simulink model "Respiratory"  (Simulink 6.4)
settings: Solver=ode45  StartTime=0.0  StopTime=10.0  RelTol=1e-3
values from neighbouring files (symbols this model uses):
  a1 = 0.3836    [Dissociation_Spencer_IC.m]    (also in Gas_Exchange_IC.m; Respiratory_IC.m)
  a2 = 1.819    [Dissociation_Spencer_IC.m]    (also in Gas_Exchange_IC.m; Respiratory_IC.m)
  alpha1 = 0.02598    [Dissociation_Spencer_IC.m]    (also in Gas_Exchange_IC.m; Respiratory_IC.m)
  alpha2 = 0.05591    [Dissociation_Spencer_IC.m]    (also in Gas_Exchange_IC.m; Respiratory_IC.m)
  beta1 = 0.012275    [Dissociation_Spencer_IC.m]    (also in Gas_Exchange_IC.m; Respiratory_IC.m)
  beta2 = 0.03255    [Dissociation_Spencer_IC.m]    (also in Gas_Exchange_IC.m; Respiratory_IC.m)
  C1 = 9    [Dissociation_Spencer_IC.m]    (also in Gas_Exchange_IC.m; Respiratory_IC.m)
  C2 = 87.00    (= 87)    [Dissociation_Spencer_IC.m]    (also in Gas_Exchange_IC.m; Respiratory_IC.m)
  Circadian_Period = 24    [Respiratory_IC.m]    (also in State_UA_Khoo_IC.m)
  CvCO2IC = 0.5116    [Body_Khoo_IC.m]    (also in Gas_Exchange_IC.m; Respiratory_IC.m = 0.5247)
  CvO2IC = 0.1672    [Body_Khoo_IC.m]    (also in Gas_Exchange_IC.m; Respiratory_IC.m = 0.1639)
  Dead1CO2IC = 0.1020    (= 0.102)    [Dead_Space_Khoo_IC.m]    (also in Gas_Exchange_IC.m; Respiratory_IC.m = 39.5616)
  Dead1O2IC = 149.8824    [Dead_Space_Khoo_IC.m]    (also in Gas_Exchange_IC.m; Respiratory_IC.m = 104.3637)
  Dead2CO2IC = 0.5274    [Dead_Space_Khoo_IC.m]    (also in Gas_Exchange_IC.m; Respiratory_IC.m = 39.6736)
  Dead2O2IC = 149.3923    [Dead_Space_Khoo_IC.m]    (also in Gas_Exchange_IC.m; Respiratory_IC.m = 104.2258)
  Dead3CO2IC = 2.2996    [Dead_Space_Khoo_IC.m]    (also in Gas_Exchange_IC.m; Respiratory_IC.m = 39.8127)
  Dead3O2IC = 147.3503    [Dead_Space_Khoo_IC.m]    (also in Gas_Exchange_IC.m; Respiratory_IC.m = 104.0505)
  Dead4CO2IC = 8.2293    [Dead_Space_Khoo_IC.m]    (also in Gas_Exchange_IC.m; Respiratory_IC.m = 40.0061)
  Dead4O2IC = 140.5179    [Dead_Space_Khoo_IC.m]    (also in Gas_Exchange_IC.m; Respiratory_IC.m = 103.8005)
  Dead5CO2IC = 22.0757    [Dead_Space_Khoo_IC.m]    (also in Gas_Exchange_IC.m; Respiratory_IC.m = 40.3359)
  Dead5O2IC = 124.5641    [Dead_Space_Khoo_IC.m]    (also in Gas_Exchange_IC.m; Respiratory_IC.m = 103.3579)
  E_CW = 5    [Pleural_Schuessler_IC.m]    (also in Pmus_Flow_Younes_IC.m; Resp_Mech_IC.m; Respiratory_IC.m)
  E_L = 5    [Pleural_Schuessler_IC.m]    (also in Pmus_Flow_Younes_IC.m; Resp_Mech_IC.m; Respiratory_IC.m)
  fc = 0.4/60    (= 0.00666666666667)    [Respiratory_IC.m]    (also in State_UA_Khoo_IC.m)
  FlowIC = 0    [Pmus_Flow_Younes_IC.m]    (also in Resp_Mech_IC.m; Respiratory_IC.m)
  gc = 0.008/60    (= 0.000133333333333)    [Respiratory_IC.m]    (also in State_UA_Khoo_IC.m)
  h = 0.0183    [Brain_Khoo_IC.m]    (also in Gas_Exchange_IC.m; Respiratory_IC.m)
  K1 = 13    [Dissociation_Spencer_IC.m]    (also in Gas_Exchange_IC.m; Respiratory_IC.m)
  K2 = 194.4    [Dissociation_Spencer_IC.m]    (also in Gas_Exchange_IC.m; Respiratory_IC.m)
  MRbCO2 = 0.0517    [Brain_Khoo_IC.m]    (also in Gas_Exchange_IC.m; Respiratory_IC.m)
  MRCO2 = 0.0033    [Body_Khoo_IC.m]    (also in Gas_Exchange_IC.m; Respiratory_IC.m)
  MRO2 = 0.0038    [Body_Khoo_IC.m]    (also in Gas_Exchange_IC.m; Respiratory_IC.m)
  PACO2_delayIC = 39.6041    [Cardio_Mix_Lange_IC.m]    (also in Gas_Exchange_IC.m; Respiratory_IC.m = 40.4448)
  PaCO2firstIC = 0.2150    (= 0.215)    [Cardio_Mix_Lange_IC.m]    (also in Gas_Exchange_IC.m; Respiratory_IC.m = -0.2465)
  PACO2IC = 37.1484    [Gas_Exchange_IC.m]    (also in Lungs_Khoo_IC.m; Respiratory_IC.m = 40.9432)
  PaCO2secondIC = 38.4577    [Cardio_Mix_Lange_IC.m]    (also in Gas_Exchange_IC.m; Respiratory_IC.m = 40.3928)
  PAO2_delayIC = 103.8436    [Cardio_Mix_Lange_IC.m]    (also in Gas_Exchange_IC.m; Respiratory_IC.m = 103.1223)
  PaO2firstIC = -0.2838    [Cardio_Mix_Lange_IC.m]    (also in Gas_Exchange_IC.m; Respiratory_IC.m = 0.3557)
  PAO2IC = 107.1983    [Gas_Exchange_IC.m]    (also in Lungs_Khoo_IC.m; Respiratory_IC.m = 102.5153)
  PaO2secondIC = 105.4828    [Cardio_Mix_Lange_IC.m]    (also in Gas_Exchange_IC.m; Respiratory_IC.m = 103.1435)
  PbCO2IC = 48.2858    [Brain_Khoo_IC.m]    (also in Gas_Exchange_IC.m; Respiratory_IC.m = 48.5383)
  PICO2 = 0    [Dead_Space_Khoo_IC.m]    (also in Gas_Exchange_IC.m; Respiratory_IC.m)
  PICO2_change = 0    [Respiratory_IC.m]
  PIO2 = 150    [Dead_Space_Khoo_IC.m]    (also in Gas_Exchange_IC.m; Respiratory_IC.m)
  PIO2_change = -90    [Mech_vent_test.m]    (also in Respiratory_IC.m = 0)
  Pt_frcIC1 = 0    [Pmus_Flow_Younes_IC.m]    (also in Resp_Mech_IC.m; Respiratory_IC.m)
  Pt_frcIC2 = 0    [Pmus_Flow_Younes_IC.m]    (also in Resp_Mech_IC.m; Respiratory_IC.m)
  QdBo = 0.8333    [Brain_Khoo_IC.m]    (also in Gas_Exchange_IC.m; Respiratory_IC.m)
  R_AW = 1.27    [Pleural_Schuessler_IC.m]    (also in Pmus_Flow_Younes_IC.m; Resp_Mech_IC.m; Respiratory_IC.m)
  R_CW = 1.03    [Pleural_Schuessler_IC.m]    (also in Pmus_Flow_Younes_IC.m; Resp_Mech_IC.m; Respiratory_IC.m)
  R_L = 1.69    [Pleural_Schuessler_IC.m]    (also in Pmus_Flow_Younes_IC.m; Resp_Mech_IC.m; Respiratory_IC.m)
  RC = 0.06    [Pleural_Schuessler_IC.m]    (also in Pmus_Flow_Younes_IC.m; Resp_Mech_IC.m; Respiratory_IC.m)
  rc = 0.2/60    (= 0.00333333333333)    [Respiratory_IC.m]    (also in State_UA_Khoo_IC.m)
  SbCO2 = 0.3600    (= 0.36)    [Brain_Khoo_IC.m]    (also in Gas_Exchange_IC.m; Respiratory_IC.m)
  SCO2 = 0.0043    [Brain_Khoo_IC.m]    (also in Gas_Exchange_IC.m; Respiratory_IC.m)
  SWAo = 0.007    [Respiratory_IC.m]    (also in State_UA_Khoo_IC.m)
  T1 = 1    [Cardio_Mix_Lange_IC.m]    (also in Gas_Exchange_IC.m; Respiratory_IC.m)
  T2 = 2    [Cardio_Mix_Lange_IC.m]    (also in Gas_Exchange_IC.m; Respiratory_IC.m)
  t_CO2_duration = 0    [Respiratory_IC.m]
  t_CO2_start = 0    [Respiratory_IC.m]
  t_end_UA = 0    [Respiratory_IC.m]    (also in State_UA_Khoo_IC.m)
  t_O2_duration = 0    [Mech_vent_test.m]    (also in Respiratory_IC.m)
  t_O2_start = 0    [Mech_vent_test.m]    (also in Respiratory_IC.m)
  t_start_UA = 0    [Respiratory_IC.m]    (also in State_UA_Khoo_IC.m)
  time_step = time_step    [acquire_data.m]    (also in acquire_data_save.m)
  VC = 5    [Pmus_Flow_Younes_IC.m]    (also in Resp_Mech_IC.m; Respiratory_IC.m)
  Vdead1 = 0.03    [Dead_Space_Khoo_IC.m]    (also in Gas_Exchange_IC.m; Respiratory_IC.m)
  Vdead2 = 0.03    [Dead_Space_Khoo_IC.m]    (also in Gas_Exchange_IC.m; Respiratory_IC.m)
  Vdead3 = 0.03    [Dead_Space_Khoo_IC.m]    (also in Gas_Exchange_IC.m; Respiratory_IC.m)
  Vdead4 = 0.03    [Dead_Space_Khoo_IC.m]    (also in Gas_Exchange_IC.m; Respiratory_IC.m)
  Vdead5 = 0.03    [Dead_Space_Khoo_IC.m]    (also in Gas_Exchange_IC.m; Respiratory_IC.m)
  VTCO2 = 15    [Body_Khoo_IC.m]    (also in Gas_Exchange_IC.m; Respiratory_IC.m)
  VtIC = 0    [Pmus_Flow_Younes_IC.m]    (also in Resp_Mech_IC.m; Respiratory_IC.m)
  VTO2 = 6    [Body_Khoo_IC.m]    (also in Gas_Exchange_IC.m; Respiratory_IC.m)
  Z = 0.0227    [Dissociation_Spencer_IC.m]    (also in Gas_Exchange_IC.m; Respiratory_IC.m)
undefined symbols (not defined in the file or in its folder): A_0_ua, Arousal_UAIC, b_ua, C_ua_awake, DAY, K_ua, R_LAW, R_trachea
libraries: simulink x1, simulink_extras x1
(part 1 of 2)
settings Model: LastModifiedBy=cPhonix
settings OptimizationCC: BlockReduction=off  BooleanDataType=off
settings DebuggingCC: SolverPrmCheckMsg=none  StrictBusMsg=None
settings HardwareCC: TargetUnknown=on

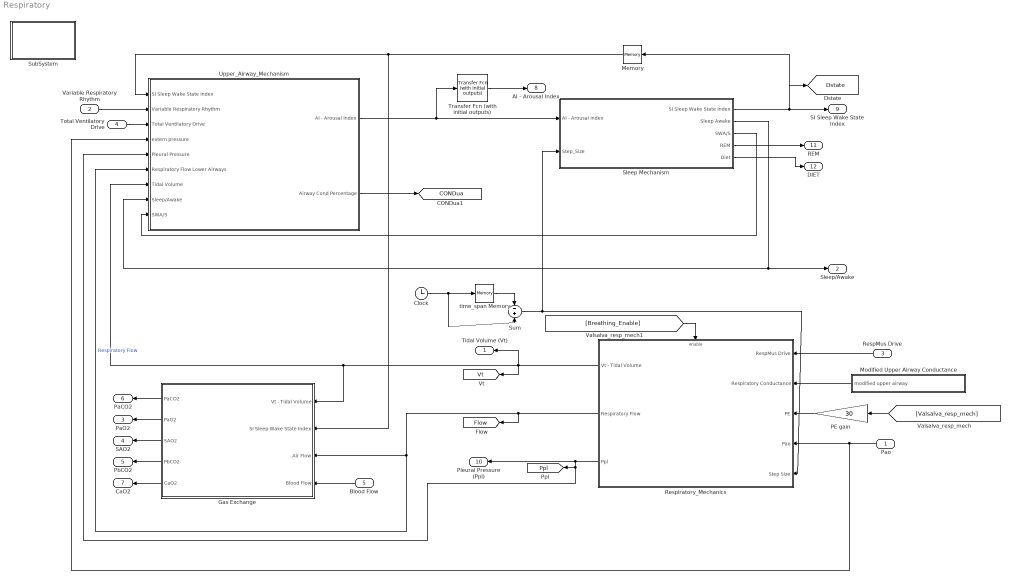
== system Respiratory ==
  Pao : Inport  Orientation=left
  Variable Respiratory Rhythm : Inport  Port=2
  RespMus Drive : Inport  Orientation=left  Port=3
  Total Ventilatory Drive : Inport  Port=4
  Blood Flow : Inport  Orientation=left  Port=5
  Clock : Clock
      settings: Decimation=10
  Gas Exchange : Subsystem  Orientation=left
  Memory : Memory  Orientation=left  InheritSampleTime=on
  Modified Upper Airway Conductance : Subsystem  Orientation=left
  PE gain : Gain  Orientation=left  Gain=30  SaturateOnIntegerOverflow=on
  Respiratory_Mechanics : Subsystem  Orientation=left  TreatAsAtomicUnit=on
      settings: PropExecContextOutsideSubsystem=on
  Sleep Mechanism : Subsystem
  SubSystem : Subsystem
      settings: OpenFcn=pneuma_variables
      mask Display: disp('"double click here"\n to load \nRespiratory \ninitial values');
  Sum : Sum  Inputs=-+  SaturateOnIntegerOverflow=on  InputSameDT=on
  Transfer Fcn (with initial outputs) : simulink_extras/Additional Linear/Transfer Fcn (with initial outputs)  SystemSampleTime=-1  N=1  D=[5 1]  Y0=Arousal_CardIC  U0=Arousal_CardIC
  Upper_Airway_Mechanism : Subsystem
  time_span Memory : Memory  X0=0-time_step
  Tidal Volume (Vt) : Outport  Orientation=left
  Sleep/Awake : Outport  Port=2
  PaO2 : Outport  Orientation=left  Port=3
  SAO2 : Outport  Orientation=left  Port=4
  PbCO2 : Outport  Orientation=left  Port=5
  PaCO2 : Outport  Orientation=left  Port=6
  CaO2 : Outport  Orientation=left  Port=7
  AI - Arousal Index : Outport  Port=8
  SI Sleep Wake State Index : Outport  Port=9
  Pleural Pressure (Ppl) : Outport  Orientation=left  Port=10
  REM : Outport  Port=11
  DIET : Outport  Port=12
  tag scope: CONDua=global, Dstate=global, Flow=global, Ppl=global, Vt=global
  wires:
  Respiratory_Mechanics/2(Respiratory Flow) -> Upper_Airway_Mechanism/6(Respiratory Flow Lower Airways), Gas Exchange/3(Air Flow), [Flow]  "Respiratory Flow"
  RespMus Drive/1 -> Respiratory_Mechanics/1("RespMus Drive ")
  PE gain/1 -> Respiratory_Mechanics/3("PE ")
  Total Ventilatory Drive/1 -> Upper_Airway_Mechanism/3(Total Ventilatory Drive)
  Modified Upper Airway Conductance/1(modified upper airway) -> Respiratory_Mechanics/2(Respiratory Conductance)
  Respiratory_Mechanics/1(Vt - Tidal Volume) -> Gas Exchange/1(Vt - Tidal Volume), Upper_Airway_Mechanism/7(Tidal Volume), Tidal Volume (Vt)/1, [Vt]
  Respiratory_Mechanics/3("Ppl ") -> Pleural Pressure (Ppl)/1, [Ppl], Upper_Airway_Mechanism/5(Pleural Pressure)
  Upper_Airway_Mechanism/1(AI - Arousal Index) -> Sleep Mechanism/1(AI - Arousal Index), Transfer Fcn (with initial outputs)/1
  Memory/1 -> Upper_Airway_Mechanism/1(SI Sleep Wake State Index), Gas Exchange/2(SI Sleep Wake State Index)
  Sleep Mechanism/1(SI Sleep Wake State Index) -> Memory/1, SI Sleep Wake State Index/1, [Dstate]
  Sleep Mechanism/2(Sleep Awake) -> Upper_Airway_Mechanism/8(Sleep/Awake), Sleep/Awake/1
  Upper_Airway_Mechanism/2("Airway Cond Percentage ") -> [CONDua]
  Gas Exchange/2(PaO2) -> PaO2/1
  Gas Exchange/1(PaCO2) -> PaCO2/1
  Gas Exchange/3(SAO2) -> SAO2/1
  Gas Exchange/4(PbCO2) -> PbCO2/1
  Pao/1 -> Upper_Airway_Mechanism/4(extern pressure), Respiratory_Mechanics/4("Pao ")
  Variable Respiratory Rhythm/1 -> Upper_Airway_Mechanism/2(Variable Respiratory Rhythm)
  Blood Flow/1 -> Gas Exchange/4(Blood Flow)
  [Breathing_Enable] -> Respiratory_Mechanics/Enable
  Sleep Mechanism/3(SWA/S) -> Upper_Airway_Mechanism/9(SWA/S)
  Clock/1 -> time_span Memory/1, Sum/2
  time_span Memory/1 -> Sum/1
  Sum/1 -> Respiratory_Mechanics/5(Step Size), Sleep Mechanism/2(Step_Size)
  Transfer Fcn (with initial outputs)/1 -> AI - Arousal Index/1
  Gas Exchange/5(CaO2) -> CaO2/1
  [Valsalva_resp_mech] -> PE gain/1
  Sleep Mechanism/4(REM) -> REM/1
  Sleep Mechanism/5(Diet) -> DIET/1

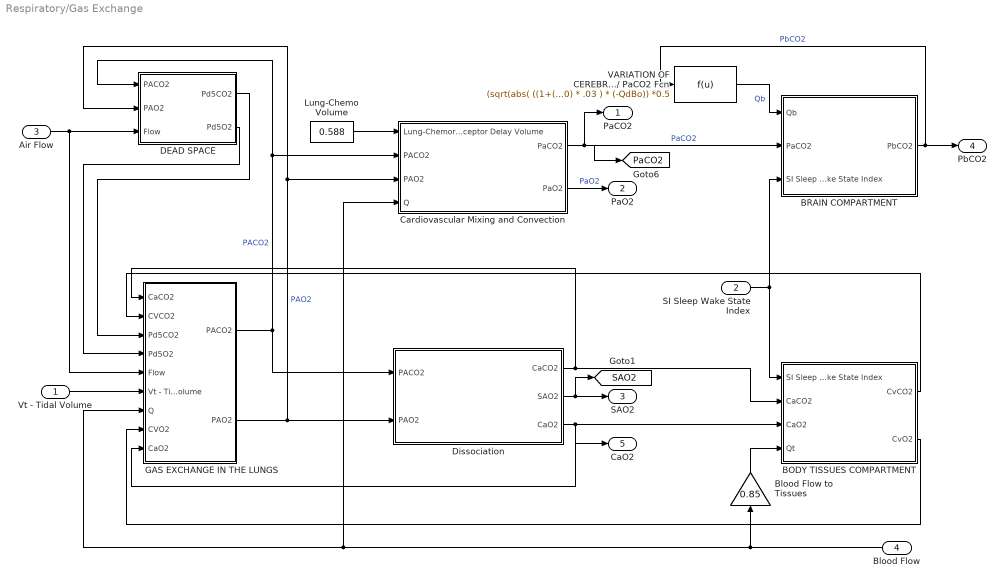
== system Respiratory/Gas Exchange ==
  Vt - Tidal Volume : Inport
  SI Sleep Wake State Index : Inport  Port=2
  Air Flow : Inport  Port=3
  Blood Flow : Inport  Orientation=left  Port=4
  BODY TISSUES COMPARTMENT : Subsystem
  BRAIN COMPARTMENT : Subsystem
  Blood Flow to Tissues : Gain  Orientation=up  Gain=0.85  SaturateOnIntegerOverflow=on
  Cardiovascular Mixing and Convection : Subsystem
  DEAD SPACE : Subsystem
  Dissociation : Subsystem
  GAS EXCHANGE IN THE LUNGS : Subsystem
  Lung-Chemo Volume : Constant  Value=0.588  OutDataType=sfix(16)  ConRadixGroup=Use specified scaling  OutScaling=2^0  SampleTime=inf  FramePeriod=inf
  VARIATION OF CEREBRAL BLOOD FLOW W/ PaCO2 Fcn : Fcn  Expr=(sqrt(abs( ((1+(u - 40) * .03 ) * (-QdBo))^2 - ( MRbCO2-h) * 4*0.03*QdBo/SCO2 ) )- (1+(u - 40) * .03 ) * (-QdBo)) *0.5
  PaCO2 : Outport
  PaO2 : Outport  Port=2
  SAO2 : Outport  Port=3
  PbCO2 : Outport  Port=4
  CaO2 : Outport  Port=5
  tag scope: PaCO2=global, SAO2=global
  wires:
  SI Sleep Wake State Index/1 -> BODY TISSUES COMPARTMENT/1(SI Sleep Wake State Index), BRAIN COMPARTMENT/3(SI Sleep Wake State Index)
  Cardiovascular Mixing and Convection/1(PaCO2) -> PaCO2/1, BRAIN COMPARTMENT/2(PaCO2), [PaCO2]  "PaCO2"
  BRAIN COMPARTMENT/1(PbCO2) -> PbCO2/1, VARIATION OF CEREBRAL BLOOD FLOW W/ PaCO2 Fcn/1  "PbCO2"
  DEAD SPACE/1(Pd5CO2) -> GAS EXCHANGE IN THE LUNGS/3(Pd5CO2)
  DEAD SPACE/2(Pd5O2) -> GAS EXCHANGE IN THE LUNGS/4(Pd5O2)
  GAS EXCHANGE IN THE LUNGS/2(PAO2) -> DEAD SPACE/2(PAO2), Cardiovascular Mixing and Convection/3(PAO2), Dissociation/2(PAO2)  "PAO2"
  Vt - Tidal Volume/1 -> GAS EXCHANGE IN THE LUNGS/6(Vt - Tidal Volume)
  Air Flow/1 -> DEAD SPACE/3(Flow), GAS EXCHANGE IN THE LUNGS/5(Flow)
  VARIATION OF CEREBRAL BLOOD FLOW W/ PaCO2 Fcn/1 -> BRAIN COMPARTMENT/1(Qb)  "Qb"
  GAS EXCHANGE IN THE LUNGS/1(PACO2) -> DEAD SPACE/1(PACO2), Cardiovascular Mixing and Convection/2(PACO2), Dissociation/1(PACO2)  "PACO2"
  Lung-Chemo Volume/1 -> Cardiovascular Mixing and Convection/1(Lung-Chemoreceptor Delay Volume)
  Blood Flow/1 -> Blood Flow to Tissues/1, GAS EXCHANGE IN THE LUNGS/7("Q "), Cardiovascular Mixing and Convection/4(Q)
  Cardiovascular Mixing and Convection/2(PaO2) -> PaO2/1  "PaO2"
  Blood Flow to Tissues/1 -> BODY TISSUES COMPARTMENT/4("Qt ")
  Dissociation/1(CaCO2) -> GAS EXCHANGE IN THE LUNGS/1(CaCO2), BODY TISSUES COMPARTMENT/2(CaCO2)
  Dissociation/3(CaO2) -> GAS EXCHANGE IN THE LUNGS/9(CaO2), CaO2/1, BODY TISSUES COMPARTMENT/3(CaO2)
  Dissociation/2(SAO2) -> [SAO2], SAO2/1
  BODY TISSUES COMPARTMENT/1(CvCO2) -> GAS EXCHANGE IN THE LUNGS/2(CVCO2)
  BODY TISSUES COMPARTMENT/2(CvO2) -> GAS EXCHANGE IN THE LUNGS/8(CVO2)

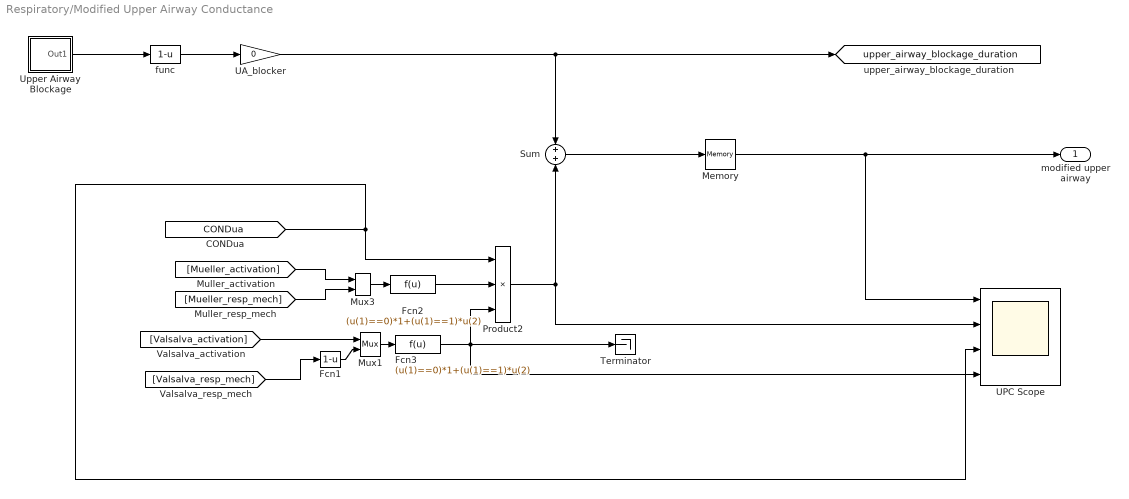
== system Respiratory/Modified Upper Airway Conductance ==
  Fcn1 : Fcn  Expr=1-u
  Fcn2 : Fcn  Expr=(u(1)==0)*1+(u(1)==1)*u(2)
  Fcn3 : Fcn  Expr=(u(1)==0)*1+(u(1)==1)*u(2)
  Memory : Memory
  Mux1 : Mux  Inputs=2
  Mux3 : Mux  Inputs=2
  Product2 : Product  Inputs=***  SaturateOnIntegerOverflow=on  InputSameDT=on
  Sum : Sum
  Terminator : Terminator
  UA_blocker : Gain  Gain=0  SaturateOnIntegerOverflow=on
  UPC Scope : Scope  NumInputPorts=4
      settings: TimeRange=120  YMin=-0.05~-0.05~0.4~-0.05  YMax=1.025~1.025~1.025~1.05  SaveName=ScopeData13  MaxDataPoints=50
  Upper Airway Blockage : Subsystem  mask{begin_time=t_start_UA, end_time=t_end_UA}
      mask prompts: begin_time "pulse begin"; end_time "pulse end"
      mask Display: disp('pulse')
  func : Fcn  Expr=1-u
  modified upper airway : Outport
  tag scope: upper_airway_blockage_duration=global
  wires:
  Upper Airway Blockage/1(Out1) -> func/1
  [Valsalva_resp_mech] -> Fcn1/1
  UA_blocker/1 -> [upper_airway_blockage_duration], Sum/1
  [CONDua] -> Product2/1, UPC Scope/3
  Product2/1 -> UPC Scope/2, Sum/2
  func/1 -> UA_blocker/1
  [Mueller_activation] -> Mux3/1
  [Mueller_resp_mech] -> Mux3/2
  Mux3/1 -> Fcn2/1
  Fcn2/1 -> Product2/2
  [Valsalva_activation] -> Mux1/1
  Mux1/1 -> Fcn3/1
  Fcn1/1 -> Mux1/2
  Fcn3/1 -> UPC Scope/4, Terminator/1, Product2/3
  Memory/1 -> modified upper airway/1, UPC Scope/1
  Sum/1 -> Memory/1

== system Respiratory/Respiratory_Mechanics ==
  "RespMus Drive " : Inport
  Respiratory Conductance : Inport  Port=2
  "PE " : Inport  Port=3
  "Pao " : Inport  Port=4
  Step Size : Inport  Port=5
  Enable : EnablePort  StatesWhenEnabling=reset  ZeroCross=off
  External Pressure Gain : Gain  Gain=0.1  SaturateOnIntegerOverflow=on
  Pleural Pressure Saturation : Saturate  UpperLimit=160  LowerLimit=-40  LinearizeAsGain=off  ZeroCross=off
  Pleural_Pressure1 : Subsystem
  Respiratory Muscles Activity1 : Subsystem
  Vt - Tidal Volume : Outport  InitialOutput=[0]
  Respiratory Flow : Outport  Port=2  InitialOutput=[0]
  "Ppl " : Outport  Port=3  InitialOutput=[0]
  wires:
  "PE "/1 -> Respiratory Muscles Activity1/2(PE)
  "RespMus Drive "/1 -> Respiratory Muscles Activity1/1(RespMus Drive)
  Respiratory Conductance/1 -> Respiratory Muscles Activity1/3("cond ")
  Respiratory Muscles Activity1/3(Pmus) -> Pleural_Pressure1/3(Pmus)
  "Pao "/1 -> External Pressure Gain/1
  External Pressure Gain/1 -> Pleural_Pressure1/4("Pao "), Respiratory Muscles Activity1/5(Pao)
  Respiratory Muscles Activity1/2(Vt) -> Pleural_Pressure1/2(Vt), Vt - Tidal Volume/1  "Vt Tidal Volume"
  Respiratory Muscles Activity1/1(Respiratory Flow) -> Pleural_Pressure1/1(Respiratory Flow), Respiratory Flow/1  "Flow"
  Step Size/1 -> Respiratory Muscles Activity1/4(Step Size)
  Pleural_Pressure1/1("Pleural Pressure (Ppl) ") -> Pleural Pressure Saturation/1
  Pleural Pressure Saturation/1 -> "Ppl "/1

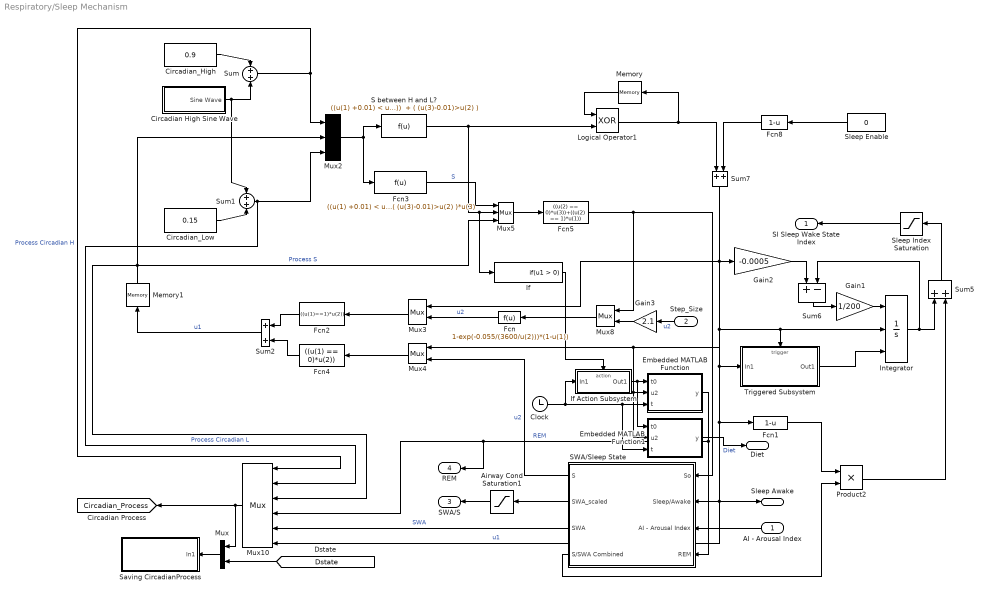
== system Respiratory/Sleep Mechanism ==
  AI - Arousal Index : Inport  Orientation=left
  Step_Size : Inport  Orientation=left  Port=2
  Airway Cond Saturation1 : Saturate  Orientation=left  UpperLimit=1  LowerLimit=0
  Circadian High Sine Wave : Subsystem
  Circadian_High : Constant  Value=0.9  OutDataType=sfix(16)  ConRadixGroup=Use specified scaling  OutScaling=2^0  SampleTime=inf  FramePeriod=inf
  Circadian_Low : Constant  Value=0.15  OutDataType=sfix(16)  ConRadixGroup=Use specified scaling  OutScaling=2^0  SampleTime=inf  FramePeriod=inf
  Clock : Clock
      settings: Decimation=10
  Embedded MATLAB Function : Stateflow chart
  Embedded MATLAB Function1 : Stateflow chart
  Fcn : Fcn  Orientation=left  Expr=1-exp(-0.055/(3600/u(2)))*(1-u(1))
  Fcn1 : Fcn  Expr=1-u
  Fcn2 : Fcn  Orientation=left  Expr=((u(1)==1)*u(2))
  Fcn3 : Fcn  Expr=((u(1) +0.01) < u(2)) * u(1) + ( (u(3)-0.01)>u(2) )*u(3)
  Fcn4 : Fcn  Orientation=left  Expr=((u(1) == 0)*u(2))
  Fcn5 : Fcn  Expr=((u(2) == 0)*u(3))+((u(2) == 1)*u(1))
  Fcn8 : Fcn  Orientation=left  Expr=1-u
  Gain1 : Gain  Gain=1/200  SaturateOnIntegerOverflow=on
  Gain2 : Gain  Gain=-0.0005  SaturateOnIntegerOverflow=on
  Gain3 : Gain  Orientation=left  Gain=2.1  SaturateOnIntegerOverflow=on
  If : If  ShowElse=off
  If Action Subsystem : Subsystem  TreatAsAtomicUnit=on
  Integrator : Integrator  ExternalReset=rising  InitialConditionSource=external  InitialCondition=1
  Logical Operator1 : Logic  Operator=XOR
  Memory : Memory  Orientation=left  X0=1  InheritSampleTime=on
  Memory1 : Memory  Orientation=up  X0=1  InheritSampleTime=on
  Mux{,3..4,8} (4 alike) : Mux  Orientation=left  Inputs=2
  Mux10 : Mux  Orientation=left  Inputs=6
  Mux2 : Mux  Inputs=3
  Mux5 : Mux  Inputs=3
  Product2 : Product  SaturateOnIntegerOverflow=on  InputSameDT=on
  S between H and L? : Fcn  Expr="((u(1) +0.01) < u(2))  + ( (u(3)-0.01)>u(2) )"
  SWA/Sleep State : Subsystem  Orientation=left
  Saving CircadianProcess : Subsystem  Orientation=left
  Sleep Enable : Constant  Orientation=left  Value=0  OutDataType=sfix(16)  ConRadixGroup=Use specified scaling  OutScaling=2^0  SampleTime=inf  FramePeriod=inf
  Sleep Index Saturation : Saturate  Orientation=left  UpperLimit=1  LowerLimit=0
  Sum : Sum  SaturateOnIntegerOverflow=on  InputSameDT=on
  Sum1 : Sum  SaturateOnIntegerOverflow=on  InputSameDT=on
  Sum2 : Sum  Orientation=left  SaturateOnIntegerOverflow=on  InputSameDT=on
  Sum5 : Sum  Orientation=up  SaturateOnIntegerOverflow=on  InputSameDT=on
  Sum6 : Sum  Orientation=down  Inputs=+-  SaturateOnIntegerOverflow=on  InputSameDT=on
  Sum7 : Sum  Orientation=down  SaturateOnIntegerOverflow=on  InputSameDT=on
  Triggered Subsystem : Subsystem  TreatAsAtomicUnit=on
  SI Sleep Wake State Index : Outport  Orientation=left
  Sleep Awake : Outport  Port=2
  SWA/S : Outport  Orientation=left  Port=3
  REM : Outport  Orientation=left  Port=4
  Diet : Outport  Port=5
  tag scope: Circadian_Process=global
  wires:
  AI - Arousal Index/1 -> SWA/Sleep State/3(AI - Arousal Index)
  Circadian_High/1 -> Sum/1
  Circadian High Sine Wave/1(Sine Wave) -> Sum/2, Sum1/1
  Circadian_Low/1 -> Sum1/2
  Sum/1 -> Mux2/1, Mux10/1  "Process Circadian H"
  Sum1/1 -> Mux2/3, Mux10/2  "Process Circadian L"
  Memory/1 -> Logical Operator1/1
  Logical Operator1/1 -> Memory/1, Sum7/1
  Fcn3/1 -> Mux5/1  "S"
  Fcn2/1 -> Sum2/1
  Sum2/1 -> Memory1/1  "u1"
  Fcn/1 -> Mux3/2  "u2"
  SWA/Sleep State/1(S) -> Mux4/2  "u2"
  Mux5/1 -> Fcn5/1
  Mux3/1 -> Fcn2/1
  Mux4/1 -> Fcn4/1
  Fcn5/1 -> SWA/Sleep State/1(So), Mux8/1
  Mux8/1 -> Fcn/1
  Step_Size/1 -> Gain3/1  "u2"
  SWA/Sleep State/2(SWA_scaled) -> Airway Cond Saturation1/1
  Airway Cond Saturation1/1 -> SWA/S/1
  Mux10/1 -> [Circadian_Process], Mux/1
  SWA/Sleep State/3(SWA) -> Mux10/5  "SWA"
  SWA/Sleep State/4(S/SWA Combined) -> Product2/2
  Fcn1/1 -> Product2/1
  Sum5/1 -> Sleep Index Saturation/1
  Product2/1 -> Sum5/2
  Sleep Index Saturation/1 -> SI Sleep Wake State Index/1
  Sum7/1 -> Gain2/1, Mux3/1, Triggered Subsystem/Trigger, Integrator/2, Fcn1/1, Sleep Awake/1, SWA/Sleep State/2(Sleep/Awake), Mux10/6, Mux4/1, Embedded MATLAB Function/2(u2), Embedded MATLAB Function1/2(u2), Triggered Subsystem/1(In1)  "u1"
  Integrator/1 -> Sum5/1, Sum6/2
  Triggered Subsystem/1(Out1) -> Integrator/3
  Gain2/1 -> Sum6/1
  Sum6/1 -> Gain1/1
  Gain1/1 -> Integrator/1
  Fcn8/1 -> Sum7/2
  Memory1/1 -> Mux5/3, Mux10/3, Mux2/2  "Process S"
  Mux2/1 -> Fcn3/1, S between H and L?/1
  S between H and L?/1 -> Logical Operator1/2, Mux5/2, If/1
  Gain3/1 -> Mux8/2
  If Action Subsystem/1(Out1) -> Embedded MATLAB Function/1(t0), Embedded MATLAB Function1/1(t0)
  If/1 -> If Action Subsystem/Action
  Fcn4/1 -> Sum2/2
  Clock/1 -> If Action Subsystem/1(In1), Embedded MATLAB Function/3(t), Embedded MATLAB Function1/3(t)
  Embedded MATLAB Function/1(y) -> SWA/Sleep State/4(REM), Mux10/4, REM/1  "REM"
  Sleep Enable/1 -> Fcn8/1
  [Dstate] -> Mux/2
  Mux/1 -> Saving CircadianProcess/1(In1)
  Embedded MATLAB Function1/1(y) -> Diet/1  "Diet"

== system Respiratory/SubSystem ==

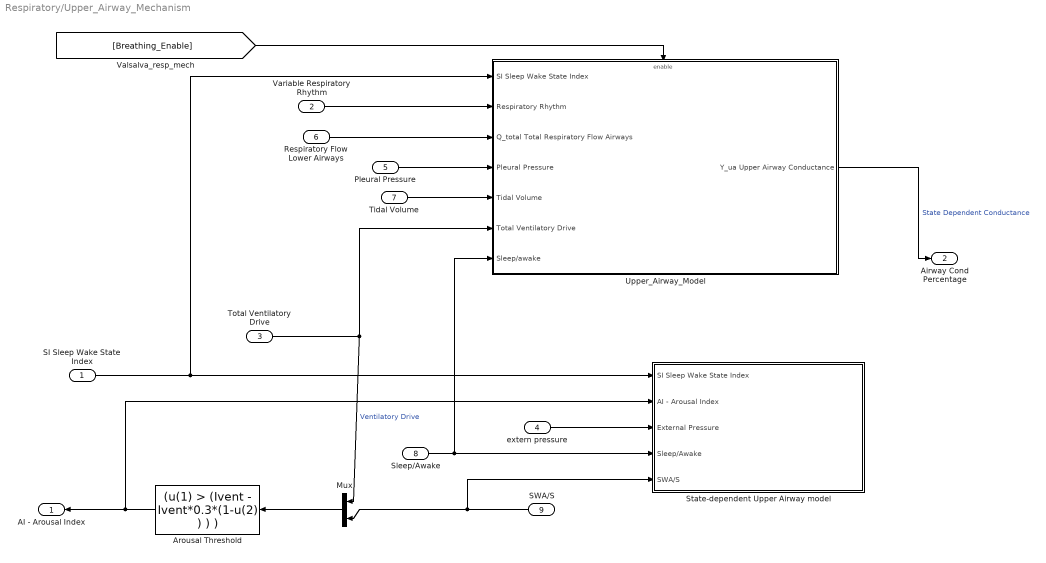
== system Respiratory/Upper_Airway_Mechanism ==
  SI Sleep Wake State Index : Inport
  Variable Respiratory Rhythm : Inport  Port=2
  Total Ventilatory Drive : Inport  Port=3
  extern pressure : Inport  Port=4
  Pleural Pressure : Inport  Port=5
  Respiratory Flow Lower Airways : Inport  Port=6
  Tidal Volume : Inport  Port=7
  Sleep/Awake : Inport  Port=8
  SWA/S : Inport  Orientation=left  Port=9
  Arousal Threshold : Fcn  Orientation=left  Expr=(u(1) > (Ivent - Ivent*0.3*(1-u(2) ) ) )
  Mux : Mux  Orientation=left  Inputs=2
  State-dependent Upper Airway model : Subsystem
  Upper_Airway_Model : Subsystem  TreatAsAtomicUnit=on
  AI - Arousal Index : Outport  Orientation=left
  "Airway Cond Percentage " : Outport  Port=2
  wires:
  SI Sleep Wake State Index/1 -> Upper_Airway_Model/1(SI Sleep Wake State Index), State-dependent Upper Airway model/1(SI Sleep Wake State Index)
  extern pressure/1 -> State-dependent Upper Airway model/3(External Pressure)
  SWA/S/1 -> Mux/2, State-dependent Upper Airway model/5(SWA/S)
  Total Ventilatory Drive/1 -> Upper_Airway_Model/6(Total Ventilatory Drive), Mux/1  "Ventilatory Drive"
  Sleep/Awake/1 -> State-dependent Upper Airway model/4(Sleep/Awake), Upper_Airway_Model/7(Sleep/awake)
  Upper_Airway_Model/1("Y_ua Upper Airway Conductance ") -> "Airway Cond Percentage "/1  "State Dependent Conductance"
  Variable Respiratory Rhythm/1 -> Upper_Airway_Model/2(Respiratory Rhythm)
  Respiratory Flow Lower Airways/1 -> Upper_Airway_Model/3(Q_total Total Respiratory Flow Airways)
  Pleural Pressure/1 -> Upper_Airway_Model/4(Pleural Pressure)
  Tidal Volume/1 -> Upper_Airway_Model/5(Tidal Volume)
  [Breathing_Enable] -> Upper_Airway_Model/Enable
  Mux/1 -> Arousal Threshold/1
  Arousal Threshold/1 -> AI - Arousal Index/1, State-dependent Upper Airway model/2(AI - Arousal Index)

== system Respiratory/Gas Exchange/BODY TISSUES COMPARTMENT ==
  SI Sleep Wake State Index : Inport  Orientation=left
  CaCO2 : Inport  Orientation=left  Port=2
  CaO2 : Inport  Orientation=left  Port=3
  "Qt " : Inport  Orientation=left  Port=4
  Body Tissues Compartment for CO2 : Subsystem  Orientation=left
  Body Tissues Compartment for O2 : Subsystem  Orientation=left
  CvCO2 : Outport  Orientation=left
  CvO2 : Outport  Orientation=left  Port=2
  wires:
  SI Sleep Wake State Index/1 -> Body Tissues Compartment for CO2/3(SI Sleep Wake State Index), Body Tissues Compartment for O2/2(SI Sleep Wake State Index)
  CaCO2/1 -> Body Tissues Compartment for CO2/1(CaCO2)
  CaO2/1 -> Body Tissues Compartment for O2/3(CaO2)
  Body Tissues Compartment for CO2/1(CvCO2) -> CvCO2/1
  Body Tissues Compartment for O2/1(CVO2) -> CvO2/1
  "Qt "/1 -> Body Tissues Compartment for O2/1(Qt), Body Tissues Compartment for CO2/2(Qt)

== system Respiratory/Gas Exchange/BRAIN COMPARTMENT ==
  Qb : Inport
  PaCO2 : Inport  Port=2
  SI Sleep Wake State Index : Inport  Port=3
  Fcn : Fcn  Expr=MRbCO2*(0.375*(1-0.4*u)+0.625)
  Fcn -5 blocks : Fcn  Expr=(u(1) + ( u(2) * u(3)) *SCO2- h ) /SbCO2
  Integrator : Integrator  InitialCondition=PbCO2IC
  Mux : Mux  Inputs=3
  sum : Sum  Inputs=+-  SaturateOnIntegerOverflow=on  InputSameDT=on
  PbCO2 : Outport
  tag scope: PbCO2IC=global
  wires:
  Fcn -5 blocks/1 -> Integrator/1
  PaCO2/1 -> sum/1
  Integrator/1 -> sum/2, [PbCO2IC], PbCO2/1
  SI Sleep Wake State Index/1 -> Fcn/1
  Mux/1 -> Fcn -5 blocks/1
  Fcn/1 -> Mux/1
  Qb/1 -> Mux/2
  sum/1 -> Mux/3

== system Respiratory/Gas Exchange/Cardiovascular Mixing and Convection ==
  Lung-Chemoreceptor Delay Volume : Inport
  PACO2 : Inport  Port=2
  PAO2 : Inport  Port=3
  Q : Inport  Port=4
  CO2 Cardiovascular Mixing and Convection Effects : Subsystem
  O2 Cardiovascular Mixing and Convection Effects : Subsystem
  PaCO2 : Outport
  PaO2 : Outport  Port=2
  wires:
  CO2 Cardiovascular Mixing and Convection Effects/1(PaCO2) -> PaCO2/1
  PACO2/1 -> CO2 Cardiovascular Mixing and Convection Effects/1(PACO2)
  Q/1 -> CO2 Cardiovascular Mixing and Convection Effects/2(Q), O2 Cardiovascular Mixing and Convection Effects/1(Q)
  Lung-Chemoreceptor Delay Volume/1 -> CO2 Cardiovascular Mixing and Convection Effects/3(Lung-Chemoreceptor Delay Volume), O2 Cardiovascular Mixing and Convection Effects/3(Lung-Chemoreceptor Delay Volume)
  O2 Cardiovascular Mixing and Convection Effects/1(PaO2) -> PaO2/1
  PAO2/1 -> O2 Cardiovascular Mixing and Convection Effects/2(PAO2)

== system Respiratory/Gas Exchange/DEAD SPACE ==
  PACO2 : Inport
  PAO2 : Inport  Port=2
  Flow : Inport  Port=3
  CO2 DEAD SPACE : Subsystem
  O2 DEAD SPACE : Subsystem
  Pd5CO2 : Outport
  Pd5O2 : Outport  Port=2
  wires:
  PACO2/1 -> CO2 DEAD SPACE/1(PACO2)
  PAO2/1 -> O2 DEAD SPACE/2(PAO2)
  CO2 DEAD SPACE/1(Pd5CO2) -> Pd5CO2/1
  O2 DEAD SPACE/1(Pd5O2) -> Pd5O2/1
  Flow/1 -> CO2 DEAD SPACE/2(Flow), O2 DEAD SPACE/1(Flow)

== system Respiratory/Gas Exchange/Dissociation ==
  PACO2 : Inport
  PAO2 : Inport  Port=2
  100 : Gain  Gain=100  SaturateOnIntegerOverflow=on
  C1*Z : Gain  Gain=C1*Z  SaturateOnIntegerOverflow=on
  CO2 Fcn -14 blocks : Fcn  Expr="(u(1) * (1+ u(2) * beta2)/((u(2) * alpha2 +1) * K2) )^(1/a2) / ( (u(1) * (1+ u(2) * beta2)/((1+ u(2) * alpha2 ) * K2) )^(1/a2)  +1) * C2*Z"
  Mux : Mux  Inputs=2
  O2 Fcn -13 blocks : Fcn  Expr="(u(2) * (1+ u(1) * beta1)/(( 1+u(1) * alpha1 ) * K1) )^(1/a1) / ( (u(2) * (1+ u(1) * beta1)/(( 1+u(1) * alpha1 ) * K1) )^(1/a1)   +1)"
  SAO2 Saturation : Saturate  Orientation=down  UpperLimit=5  LowerLimit=-5
  CaCO2 : Outport
  SAO2 : Outport  Port=2
  CaO2 : Outport  Port=3
  wires:
  CO2 Fcn -14 blocks/1 -> CaCO2/1
  C1*Z/1 -> CaO2/1
  O2 Fcn -13 blocks/1 -> C1*Z/1, SAO2 Saturation/1
  PACO2/1 -> Mux/1
  PAO2/1 -> Mux/2
  100/1 -> SAO2/1
  SAO2 Saturation/1 -> 100/1
  Mux/1 -> CO2 Fcn -14 blocks/1, O2 Fcn -13 blocks/1

== system Respiratory/Gas Exchange/GAS EXCHANGE IN THE LUNGS ==
  CaCO2 : Inport
  CVCO2 : Inport  Port=2
  Pd5CO2 : Inport  Port=3
  Pd5O2 : Inport  Port=4
  Flow : Inport  Port=5
  Vt - Tidal Volume : Inport  Port=6
  "Q " : Inport  Port=7
  CVO2 : Inport  Port=8
  CaO2 : Inport  Port=9
  CO2 Gas Exchange in the Lungs : Subsystem
  O2 Gas Exchange in the Lungs : Subsystem
  PACO2 : Outport
  PAO2 : Outport  Port=2
  wires:
  CO2 Gas Exchange in the Lungs/1(PACO2) -> PACO2/1
  O2 Gas Exchange in the Lungs/1(PAO2) -> PAO2/1
  CaCO2/1 -> CO2 Gas Exchange in the Lungs/1(CaCO2)
  CVCO2/1 -> CO2 Gas Exchange in the Lungs/2(CVCO2)
  Pd5CO2/1 -> CO2 Gas Exchange in the Lungs/3(Pd5CO2)
  Vt - Tidal Volume/1 -> O2 Gas Exchange in the Lungs/1(Vt - Tidal Volume), CO2 Gas Exchange in the Lungs/4(Vt - Tidal Volume)
  Flow/1 -> O2 Gas Exchange in the Lungs/2(Flow), CO2 Gas Exchange in the Lungs/5(Flow)
  "Q "/1 -> O2 Gas Exchange in the Lungs/3(Q), CO2 Gas Exchange in the Lungs/6("Q ")
  CaO2/1 -> O2 Gas Exchange in the Lungs/4(CaO2)
  CVO2/1 -> O2 Gas Exchange in the Lungs/5(CVO2)
  Pd5O2/1 -> O2 Gas Exchange in the Lungs/6(Pd5O2)

== system Respiratory/Modified Upper Airway Conductance/Upper Airway Blockage ==
  Step : Step  Time=end_time  Before=1  After=0  SampleTime=0
  Step1 : Step  Time=begin_time  SampleTime=0
  Sum : Sum  Inputs=|++  SaturateOnIntegerOverflow=on  InputSameDT=on
  Out1 : Outport
  wires:
  Sum/1 -> Out1/1
  Step1/1 -> Sum/2
  Step/1 -> Sum/1

== system Respiratory/Respiratory_Mechanics/Pleural_Pressure1 ==
  Respiratory Flow : Inport
  Vt : Inport  Port=2
  Pmus : Inport  Port=3
  "Pao " : Inport  Port=4
  Pa : Subsystem
  Pcw : Subsystem
  Sum1 : Sum  Inputs=-++  SaturateOnIntegerOverflow=on  InputSameDT=on
  "Pleural Pressure (Ppl) " : Outport
  wires:
  Sum1/1 -> "Pleural Pressure (Ppl) "/1
  Respiratory Flow/1 -> Pcw/2(Flow), Pa/1("Flow   ")
  "Pao "/1 -> Pa/2("Pao ")
  Pcw/1("Pcw  ") -> Sum1/2
  Pmus/1 -> Sum1/1
  Pa/1("Pa ") -> Sum1/3
  Vt/1 -> Pcw/1(Vt)

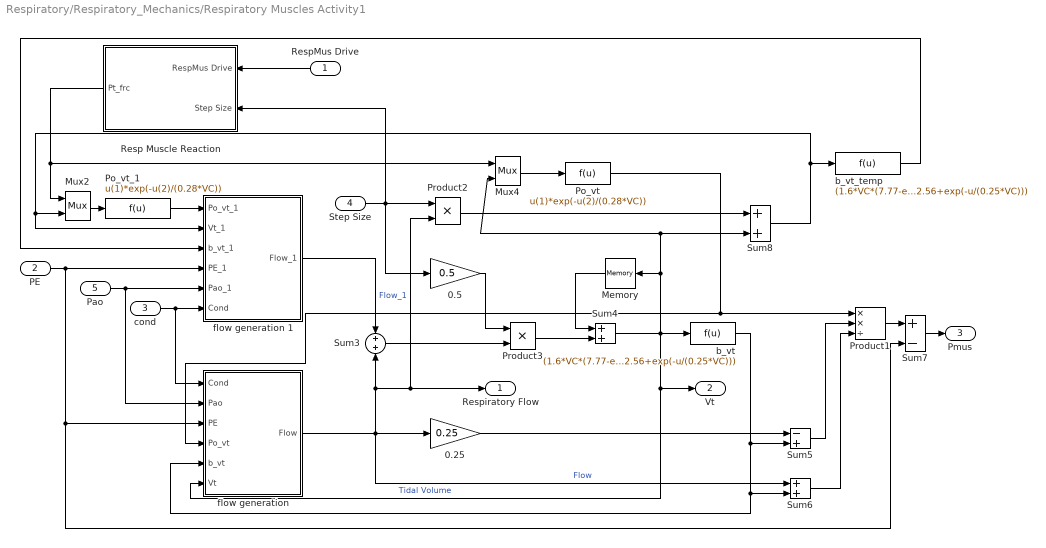
== system Respiratory/Respiratory_Mechanics/Respiratory Muscles Activity1 ==
  RespMus Drive : Inport  Orientation=left
  PE : Inport  Port=2
  "cond " : Inport  Port=3
  Step Size : Inport  Port=4
  Pao : Inport  Port=5
  0.25 : Gain  Gain=0.25  SaturateOnIntegerOverflow=on
  0.5 : Gain  Gain=0.5  SaturateOnIntegerOverflow=on
  Memory : Memory  Orientation=left  X0=VtIC  InheritSampleTime=on
  Mux2 : Mux  Inputs=2
  Mux4 : Mux  Inputs=2
  Po_vt : Fcn  Expr=u(1)*exp(-u(2)/(0.28*VC))
  Po_vt_1 : Fcn  Expr=u(1)*exp(-u(2)/(0.28*VC))
  Product1 : Product  Inputs=**/  SaturateOnIntegerOverflow=on  InputSameDT=on
  Product2 : Product  SaturateOnIntegerOverflow=on  InputSameDT=on
  Product3 : Product  SaturateOnIntegerOverflow=on  InputSameDT=on
  Resp Muscle Reaction : Subsystem  Orientation=left
  Sum{3..4,6,8} (4 alike) : Sum  SaturateOnIntegerOverflow=on  InputSameDT=on
  Sum5 : Sum  Inputs=-+  SaturateOnIntegerOverflow=on  InputSameDT=on
  Sum7 : Sum  Inputs=+-  SaturateOnIntegerOverflow=on  InputSameDT=on
  b_vt : Fcn  Expr=(1.6*VC*(7.77-exp(-u/(0.25*VC))))/(2.56+exp(-u/(0.25*VC)))
  b_vt_temp : Fcn  Expr=(1.6*VC*(7.77-exp(-u/(0.25*VC))))/(2.56+exp(-u/(0.25*VC)))
  flow generation : Subsystem
  flow generation 1 : Subsystem
  Respiratory Flow : Outport
  Vt : Outport  Port=2
  Pmus : Outport  Port=3
  wires:
  Product3/1 -> Sum4/2
  Mux2/1 -> Po_vt_1/1
  Po_vt_1/1 -> flow generation 1/1(Po_vt_1)
  Sum5/1 -> Product1/2
  Sum6/1 -> Product1/3
  Mux4/1 -> Po_vt/1
  b_vt_temp/1 -> flow generation 1/3(b_vt_1)
  flow generation 1/1(Flow_1) -> Sum3/1  "Flow_1"
  "cond "/1 -> flow generation 1/6("Cond "), flow generation/1("Cond ")
  PE/1 -> flow generation 1/4(PE_1), flow generation/3(PE), Sum7/2
  Pao/1 -> flow generation 1/5(Pao_1), flow generation/2("Pao ")
  Memory/1 -> Sum4/1
  flow generation/1(Flow) -> Sum3/2, Product2/2, Respiratory Flow/1, 0.25/1, Sum6/1  "Flow"
  Sum8/1 -> b_vt_temp/1, flow generation 1/2(Vt_1), Mux2/2
  Sum7/1 -> Pmus/1
  RespMus Drive/1 -> Resp Muscle Reaction/1(RespMus Drive)
  Product1/1 -> Sum7/1
  0.25/1 -> Sum5/1
  Sum4/1 -> Memory/1, Sum8/2, Mux4/2, flow generation/6(Vt), Vt/1, b_vt/1  "Tidal Volume"
  0.5/1 -> Product3/1
  Sum3/1 -> Product3/2
  Product2/1 -> Sum8/1
  Resp Muscle Reaction/1(Pt_frc) -> Mux2/1, Mux4/1
  Step Size/1 -> Resp Muscle Reaction/2(Step Size), Product2/1, 0.5/1
  b_vt/1 -> Sum5/2, Sum6/2, flow generation/5(b_vt)
  Po_vt/1 -> flow generation/4("Po_vt "), Product1/1

== system Respiratory/Sleep Mechanism/Circadian High Sine Wave ==
  Gain4 : Gain  Gain=0.97  SaturateOnIntegerOverflow=on
  Gain5 : Gain  Gain=0.22  SaturateOnIntegerOverflow=on
  Gain6 : Gain  Gain=0.07  SaturateOnIntegerOverflow=on
  Gain7 : Gain  Gain=0.03  SaturateOnIntegerOverflow=on
  Gain8 : Gain  Gain=0.01  SaturateOnIntegerOverflow=on
  Sin(2*theta) : Sin  Amplitude=0.12  Frequency=0.00014544  Phase=3.2358  SampleTime=0
  Sin(3*theta) : Sin  Amplitude=0.12  Frequency=0.00021817  Phase=3.2358  SampleTime=0
  Sin(4*theta) : Sin  Amplitude=0.12  Frequency=0.00029089  Phase=3.2358  SampleTime=0
  Sin(5*theta) : Sin  Amplitude=0.12  Frequency=0.00036361  Phase=3.2358  SampleTime=0
  Sin(theta) : Sin  Amplitude=0.12  Frequency=7.2722e-005  Phase=3.2358  SampleTime=0
  Sum : Sum  Inputs=|+++++  SaturateOnIntegerOverflow=on  InputSameDT=on
  Sine Wave : Outport
  wires:
  Sin(theta)/1 -> Gain4/1
  Gain4/1 -> Sum/1
  Sin(2*theta)/1 -> Gain5/1
  Gain5/1 -> Sum/2
  Sin(3*theta)/1 -> Gain6/1
  Gain6/1 -> Sum/3
  Sin(4*theta)/1 -> Gain7/1
  Gain7/1 -> Sum/4
  Sin(5*theta)/1 -> Gain8/1
  Gain8/1 -> Sum/5
  Sum/1 -> Sine Wave/1

== system Respiratory/Sleep Mechanism/If Action Subsystem ==
  In1 : Inport
  Action Port : ActionPort
  Out1 : Outport
  wires:
  In1/1 -> Out1/1

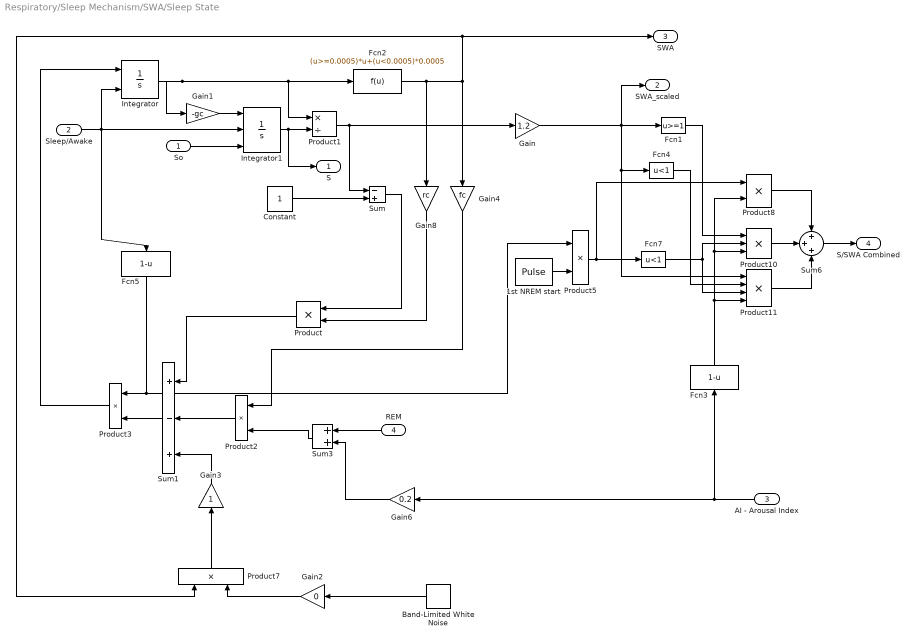
== system Respiratory/Sleep Mechanism/SWA/Sleep State ==
  So : Inport
  Sleep/Awake : Inport  Port=2
  AI - Arousal Index : Inport  Orientation=left  Port=3
  REM : Inport  Orientation=left  Port=4
  1st NREM start : DiscretePulseGenerator  PulseType=Time based  Period=Circadian_Period*3600  PulseWidth=100 - 85 *1.8 /Circadian_Period  PhaseDelay=3600*1.8*0.85+5
  Band-Limited White Noise : simulink/Sources/Band-Limited White Noise  Orientation=left  SystemSampleTime=-1  Cov=[0.1]  Ts=0.1  seed=[23341]
  Constant : Constant  Value=1  OutDataType=sfix(16)  ConRadixGroup=Use specified scaling  OutScaling=2^0  SampleTime=inf  FramePeriod=inf
  Fcn1 : Fcn  Expr=u>=1
  Fcn2 : Fcn  Expr=(u>=0.0005)*u+(u<0.0005)*0.0005
  Fcn3 : Fcn  Orientation=up  Expr=1-u
  Fcn4 : Fcn  Expr=u<1
  Fcn5 : Fcn  Orientation=down  Expr=1-u
  Fcn7 : Fcn  Expr=u<1
  Gain : Gain  Gain=1.2
  Gain1 : Gain  Gain=-gc  SaturateOnIntegerOverflow=on
  Gain2 : Gain  Orientation=left  Gain=0  SaturateOnIntegerOverflow=on
  Gain3 : Gain  Orientation=up  SaturateOnIntegerOverflow=on
  Gain4 : Gain  Orientation=down  Gain=fc  SaturateOnIntegerOverflow=on
  Gain6 : Gain  Orientation=left  Gain=0.2  SaturateOnIntegerOverflow=on
  Gain8 : Gain  Orientation=down  Gain=rc  SaturateOnIntegerOverflow=on
  Integrator : Integrator  ExternalReset=either  InitialCondition=SWAo  LimitOutput=on  UpperSaturationLimit=1  LowerSaturationLimit=0
  Integrator1 : Integrator  ExternalReset=falling  InitialConditionSource=external  InitialCondition=0.8  LimitOutput=on
  Product : Product  Orientation=left  SaturateOnIntegerOverflow=on  InputSameDT=on
  Product1 : Product  Inputs=*/  SaturateOnIntegerOverflow=on  InputSameDT=on
  Product10 : Product  Inputs=3  SaturateOnIntegerOverflow=on  InputSameDT=on
  Product11 : Product  Inputs=4  SaturateOnIntegerOverflow=on  InputSameDT=on
  Product2 : Product  Orientation=left  SaturateOnIntegerOverflow=on  InputSameDT=on
  Product3 : Product  Orientation=left  SaturateOnIntegerOverflow=on  InputSameDT=on
  Product5 : Product  Inputs=**  SaturateOnIntegerOverflow=on  InputSameDT=on
  Product7 : Product  Orientation=up  SaturateOnIntegerOverflow=on  InputSameDT=on
  Product8 : Product  SaturateOnIntegerOverflow=on  InputSameDT=on
  Sum : Sum  Inputs=-+  SaturateOnIntegerOverflow=on  InputSameDT=on
  Sum1 : Sum  Orientation=left  Inputs=+-+  SaturateOnIntegerOverflow=on  InputSameDT=on
  Sum3 : Sum  Orientation=left  SaturateOnIntegerOverflow=on  InputSameDT=on
  Sum6 : Sum  Inputs=+++  SaturateOnIntegerOverflow=on  InputSameDT=on
  S : Outport
  SWA_scaled : Outport  Port=2
  SWA : Outport  Port=3
  S/SWA Combined : Outport  Port=4
  wires:
  Fcn4/1 -> Product11/2
  Fcn7/1 -> Product11/3, Product10/2
  Product10/1 -> Sum6/2
  Product11/1 -> Sum6/3
  Sum6/1 -> S/SWA Combined/1
  Product8/1 -> Sum6/1
  Gain2/1 -> Product7/2
  Product7/1 -> Gain3/1
  Gain6/1 -> Sum3/2
  AI - Arousal Index/1 -> Gain6/1, Fcn3/1
  Sum3/1 -> Product2/2
  Constant/1 -> Sum/2
  Product1/1 -> Sum/1, Gain/1
  Gain1/1 -> Integrator1/1
  Integrator/1 -> Product1/1, Fcn2/1, Gain1/1
  Sum/1 -> Product/1
  Product/1 -> Sum1/1
  Product2/1 -> Sum1/2
  Gain3/1 -> Sum1/3
  Integrator1/1 -> Product1/2, S/1
  Sleep/Awake/1 -> Integrator1/2, Fcn5/1, Integrator/2
  So/1 -> Integrator1/3
  Fcn2/1 -> Gain4/1, Product7/1, SWA/1, Gain8/1
  Gain/1 -> SWA_scaled/1, Fcn1/1, Product11/1, Fcn4/1
  Gain4/1 -> Product2/1
  Gain8/1 -> Product/2
  Sum1/1 -> Product3/2
  Product3/1 -> Integrator/1
  Fcn5/1 -> Product3/1, Product5/1
  Fcn3/1 -> Product8/2, Product10/3, Product11/4
  Band-Limited White Noise/1 -> Gain2/1
  Product5/1 -> Fcn7/1, Product8/1
  1st NREM start/1 -> Product5/2
  Fcn1/1 -> Product10/1
  REM/1 -> Sum3/1

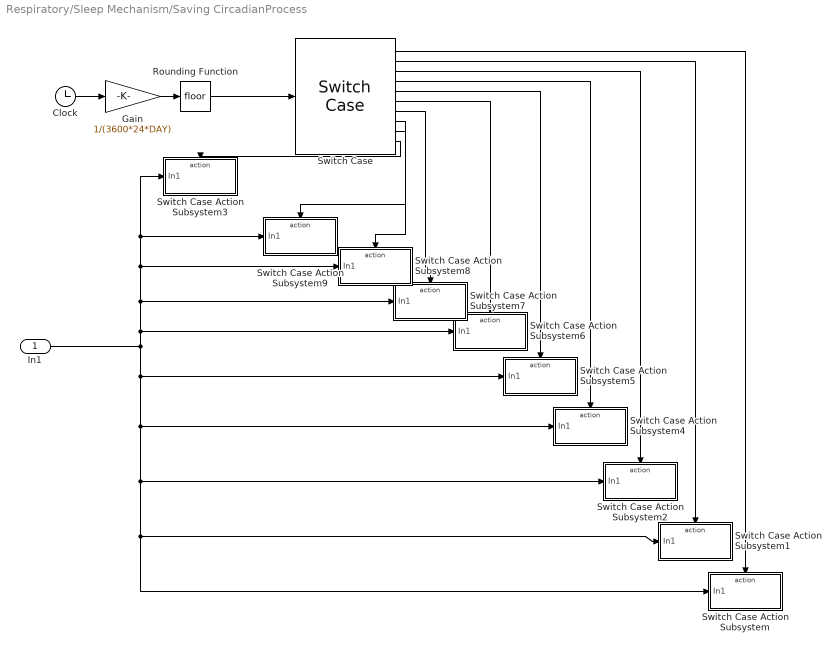
== system Respiratory/Sleep Mechanism/Saving CircadianProcess ==
  In1 : Inport
  Clock : Clock
      settings: Decimation=10
  Gain : Gain  Gain=1/(3600*24*DAY)
  Rounding Function : Rounding
  Switch Case : SwitchCase  CaseConditions={0,1,2,3,4,5,6,7,8}  SampleTime=sampletime
  Switch Case Action Subsystem : Subsystem  TreatAsAtomicUnit=on
  Switch Case Action Subsystem1 : Subsystem  TreatAsAtomicUnit=on
  Switch Case Action Subsystem2 : Subsystem  TreatAsAtomicUnit=on
  Switch Case Action Subsystem3 : Subsystem  TreatAsAtomicUnit=on
  Switch Case Action Subsystem4 : Subsystem  TreatAsAtomicUnit=on
  Switch Case Action Subsystem5 : Subsystem  TreatAsAtomicUnit=on
  Switch Case Action Subsystem6 : Subsystem  TreatAsAtomicUnit=on
  Switch Case Action Subsystem7 : Subsystem  TreatAsAtomicUnit=on
  Switch Case Action Subsystem8 : Subsystem  TreatAsAtomicUnit=on
  Switch Case Action Subsystem9 : Subsystem  TreatAsAtomicUnit=on
  wires:
  Clock/1 -> Gain/1
  Switch Case/1 -> Switch Case Action Subsystem/Action
  Switch Case/2 -> Switch Case Action Subsystem1/Action
  Switch Case/3 -> Switch Case Action Subsystem2/Action
  Switch Case/10 -> Switch Case Action Subsystem3/Action
  Rounding Function/1 -> Switch Case/1
  In1/1 -> Switch Case Action Subsystem/1(In1), Switch Case Action Subsystem1/1(In1), Switch Case Action Subsystem2/1(In1), Switch Case Action Subsystem5/1(In1), Switch Case Action Subsystem3/1(In1), Switch Case Action Subsystem9/1(In1), Switch Case Action Subsystem8/1(In1), Switch Case Action Subsystem7/1(In1), Switch Case Action Subsystem6/1(In1), Switch Case Action Subsystem4/1(In1)
  Gain/1 -> Rounding Function/1
  Switch Case/4 -> Switch Case Action Subsystem4/Action
  Switch Case/5 -> Switch Case Action Subsystem5/Action
  Switch Case/6 -> Switch Case Action Subsystem6/Action
  Switch Case/7 -> Switch Case Action Subsystem7/Action
  Switch Case/8 -> Switch Case Action Subsystem8/Action
  Switch Case/9 -> Switch Case Action Subsystem9/Action

== system Respiratory/Sleep Mechanism/Triggered Subsystem ==
  In1 : Inport
  Trigger : TriggerPort
  Out1 : Outport
  wires:
  In1/1 -> Out1/1

== system Respiratory/Upper_Airway_Mechanism/State-dependent Upper Airway model ==
  SI Sleep Wake State Index : Inport
  AI - Arousal Index : Inport  Port=2
  External Pressure : Inport  Port=3
  Sleep/Awake : Inport  Port=4
  SWA/S : Inport  Port=5
  Airway Cond Saturation2 : Saturate  UpperLimit=1  LowerLimit=0
  Fcn1 : Fcn  Expr="((u(1) >=1.0) * u(2) * (1 + 0.3 * (1 - u(3)) * (1-u(4)) )  + ( u(1)<1.0) * u(1) * u(2) ) *(1- u(5))* u(1)"
  Integrator : Integrator  ExternalReset=rising  InitialCondition=Arousal_UAIC
  Mux1 : Mux  Inputs=5
  PE gain2 : Gain  Gain=1/15  SaturateOnIntegerOverflow=on
  S_UA : Constant  Value=0.05  OutDataType=sfix(16)  ConRadixGroup=Use specified scaling  OutScaling=2^0  SampleTime=inf  FramePeriod=inf
  sum3 : Sum  Inputs=-+  SaturateOnIntegerOverflow=on  InputSameDT=on
  tag scope: Arousal_UAIC=global
  wires:
  AI - Arousal Index/1 -> Integrator/2, Mux1/5
  SI Sleep Wake State Index/1 -> Mux1/1
  SWA/S/1 -> Mux1/3
  Sleep/Awake/1 -> Mux1/4
  S_UA/1 -> sum3/2
  sum3/1 -> Airway Cond Saturation2/1
  External Pressure/1 -> PE gain2/1
  PE gain2/1 -> sum3/1
  Mux1/1 -> Fcn1/1
  Airway Cond Saturation2/1 -> Mux1/2
  Fcn1/1 -> Integrator/1
  Integrator/1 -> [Arousal_UAIC]

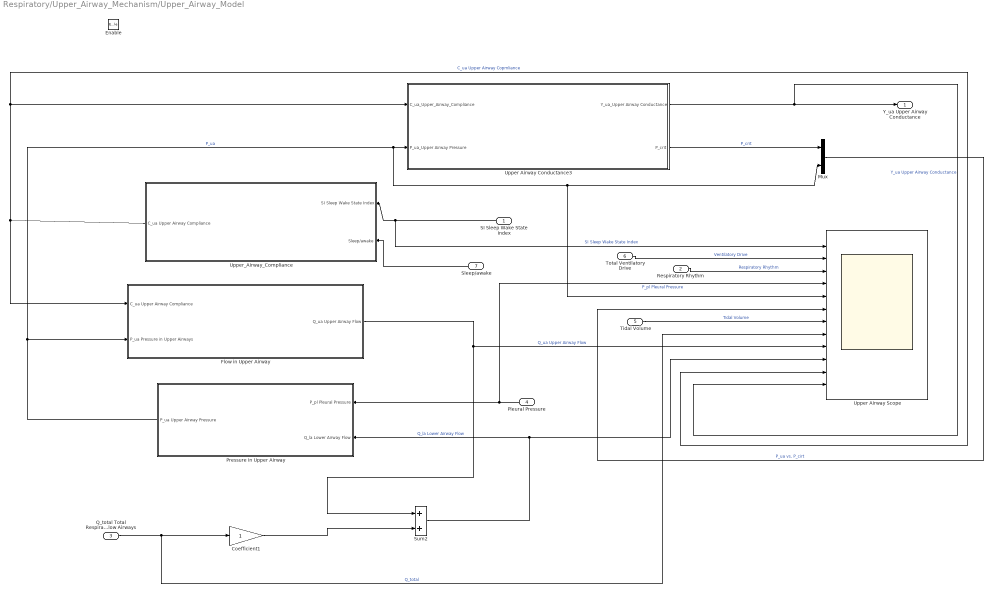
== system Respiratory/Upper_Airway_Mechanism/Upper_Airway_Model ==
  SI Sleep Wake State Index : Inport  Orientation=left
  Respiratory Rhythm : Inport  Port=2
  Q_total Total Respiratory Flow Airways : Inport  Port=3
  Pleural Pressure : Inport  Orientation=left  Port=4
  Tidal Volume : Inport  Port=5
  Total Ventilatory Drive : Inport  Port=6
  Sleep/awake : Inport  Orientation=left  Port=7
  Enable : EnablePort
  " Flow in Upper Airway" : Subsystem
  " Pressure in Upper Airway" : Subsystem  Orientation=left
  Coefficient1 : Gain  SaturateOnIntegerOverflow=on
  Mux : Mux  Inputs=2
  Sum2 : Sum  SaturateOnIntegerOverflow=on
  Upper Airway Conductance3 : Subsystem
  Upper Airway Scope : Scope  NumInputPorts=12
      settings: TimeRange=120  YMin=0~0.2~-0.05~-40~-4~-41~-0.1~-2~-2e-006~-4~0.005~0.5  YMax=1~0.48~1.05~5~1.5~10~3~2.5~5e-006~5~0.01~1.05  SaveName=ScopeData20  MaxDataPoints=50
  Upper_Airway_Compliance : Subsystem  Orientation=left
  "Y_ua Upper Airway Conductance " : Outport  InitialOutput=[0]
  wires:
  Q_total Total Respiratory Flow Airways/1 -> Upper Airway Scope/8, Coefficient1/1  "Q_total"
  SI Sleep Wake State Index/1 -> Upper_Airway_Compliance/1("SI Sleep Wake State Index "), Upper Airway Scope/1  "SI Sleep Wake State Index"
  Pleural Pressure/1 -> Upper Airway Scope/4, " Pressure in Upper Airway"/1(P_pl Pleural Pressure)  "P_pl Pleural Pressure"
  Sum2/1 -> " Pressure in Upper Airway"/2(Q_la Lower Airway Flow), Upper Airway Scope/10  "Q_la Lower Airway Flow"
  " Pressure in Upper Airway"/1("P_ua Upper Airway Pressure ") -> " Flow in Upper Airway"/2(P_ua Pressure in Upper Airways), Upper Airway Conductance3/2(P_ua_Upper Airway Pressure), Mux/2, Upper Airway Scope/5  "P_ua"
  Upper Airway Conductance3/2(P_crit) -> Mux/1  "P_crit"
  Upper_Airway_Compliance/1(C_ua Upper Airway Compliance) -> " Flow in Upper Airway"/1(C_ua Upper Airway Compliance), Upper Airway Conductance3/1(C_ua_Upper_Airway_Compliance), Upper Airway Scope/11  "C_ua Upper Airway Copmliance"
  " Flow in Upper Airway"/1("Q_ua Upper Airway Flow ") -> Upper Airway Scope/9, Sum2/1  "Q_ua Upper Airway Flow"
  Upper Airway Conductance3/1(Y_ua_Upper Airway Conductance) -> Upper Airway Scope/12, "Y_ua Upper Airway Conductance "/1  "Y_ua Upper Airway Conductance"
  Total Ventilatory Drive/1 -> Upper Airway Scope/2  "Ventilatory Drive"
  Mux/1 -> Upper Airway Scope/6  "P_ua vs. P_cirt"
  Tidal Volume/1 -> Upper Airway Scope/7  "Tidal Volume"
  Respiratory Rhythm/1 -> Upper Airway Scope/3  "Respiratory Rhythm"
  Sleep/awake/1 -> Upper_Airway_Compliance/2(Sleep/awake)
  Coefficient1/1 -> Sum2/2

== system Respiratory/Gas Exchange/BODY TISSUES COMPARTMENT/Body Tissues Compartment for CO2 ==
  CaCO2 : Inport
  Qt : Inport  Port=2
  SI Sleep Wake State Index : Inport  Port=3
  Fcn : Fcn  Expr=MRCO2*(0.375*(1-0.4*u)+0.625)
  Fcn -5 blocks : Fcn  Expr=( u(1) + ( u(2) * u(3)) ) /VTCO2
  Integrator : Integrator  InitialCondition=CvCO2IC
  Mux : Mux  Inputs=3
  Sum1 : Sum  Inputs=+-  SaturateOnIntegerOverflow=on  InputSameDT=on
  CvCO2 : Outport
  tag scope: CvCO2IC=global
  wires:
  SI Sleep Wake State Index/1 -> Fcn/1
  CaCO2/1 -> Sum1/1
  Fcn -5 blocks/1 -> Integrator/1
  Integrator/1 -> [CvCO2IC], Sum1/2, CvCO2/1
  Mux/1 -> Fcn -5 blocks/1
  Fcn/1 -> Mux/1
  Qt/1 -> Mux/2
  Sum1/1 -> Mux/3

== system Respiratory/Gas Exchange/BODY TISSUES COMPARTMENT/Body Tissues Compartment for O2 ==
  Qt : Inport
  SI Sleep Wake State Index : Inport  Port=2
  CaO2 : Inport  Port=3
  Fcn : Fcn  Expr=MRO2*(0.375*(1-0.4*u)+0.625)
  Fcn -5 blocks : Fcn  Expr=( -u(1) + ( u(2) * u(3)) ) /VTO2
  Integrator : Integrator  InitialCondition=CvO2IC
  Mux : Mux  Inputs=3
  Sum1 : Sum  Inputs=+-  SaturateOnIntegerOverflow=on  InputSameDT=on
  CVO2 : Outport
  tag scope: CvO2IC=global
  wires:
  SI Sleep Wake State Index/1 -> Fcn/1
  Qt/1 -> Mux/2
  Sum1/1 -> Mux/3
  CaO2/1 -> Sum1/1
  Fcn -5 blocks/1 -> Integrator/1
  Integrator/1 -> [CvO2IC], Sum1/2, CVO2/1
  Mux/1 -> Fcn -5 blocks/1
  Fcn/1 -> Mux/1

== system Respiratory/Gas Exchange/Cardiovascular Mixing and Convection/CO2 Cardiovascular Mixing and Convection Effects ==
  PACO2 : Inport
  Q : Inport  Port=2
  Lung-Chemoreceptor Delay Volume : Inport  Port=3
  1/(T1*T2) : Gain  Gain=1/(T1*T2)  SaturateOnIntegerOverflow=on
  Integrator : Integrator  InitialCondition=PaCO2firstIC
  Integrator1 : Integrator  InitialCondition=PaCO2secondIC
  PACO2 delay : VariableTransportDelay  MaximumDelay=100  InitialOutput=PACO2_delayIC  MaximumPoints=22528
  Product1 : Product  Inputs=*/  SaturateOnIntegerOverflow=on  InputSameDT=on
  Sum : Sum  Inputs=--+  SaturateOnIntegerOverflow=on  InputSameDT=on
  T1+T2 : Gain  Orientation=left  Gain=T1+T2  SaturateOnIntegerOverflow=on
  PaCO2 : Outport
  tag scope: PACO2_delayIC=global, PaCO2firstIC=global, PaCO2secondIC=global
  wires:
  T1+T2/1 -> Sum/1
  Integrator/1 -> T1+T2/1, Integrator1/1, [PaCO2firstIC]
  Sum/1 -> 1/(T1*T2)/1
  1/(T1*T2)/1 -> Integrator/1
  Integrator1/1 -> Sum/2, [PaCO2secondIC], PaCO2/1
  PACO2/1 -> PACO2 delay/1
  PACO2 delay/1 -> [PACO2_delayIC], Sum/3
  Product1/1 -> PACO2 delay/2
  Lung-Chemoreceptor Delay Volume/1 -> Product1/1
  Q/1 -> Product1/2

== system Respiratory/Gas Exchange/Cardiovascular Mixing and Convection/O2 Cardiovascular Mixing and Convection Effects ==
  note: Warning: Division by zero in block 'pneuma_cardiovascular/Respiratory_System/Gas Exchange/Cardiovascular Mixing and Convection/O2 Cardiovascular Mixing and Convection Effects/PAO2 Save Subsystem/Product1'.
  Q : Inport
  PAO2 : Inport  Port=2
  Lung-Chemoreceptor Delay Volume : Inport  Port=3
  1/(T1*T2) : Gain  Gain=1/(T1*T2)  SaturateOnIntegerOverflow=on
  Integrator : Integrator  InitialCondition=PaO2firstIC
  Integrator1 : Integrator  InitialCondition=PaO2secondIC
  PAO2 delay : VariableTransportDelay  MaximumDelay=100  InitialOutput=PAO2_delayIC  MaximumPoints=22528
  Product1 : Product  Inputs=*/  SaturateOnIntegerOverflow=on  InputSameDT=on
  Sum : Sum  Inputs=+--  SaturateOnIntegerOverflow=on  InputSameDT=on
  T1+T2 : Gain  Orientation=left  Gain=T1+T2  SaturateOnIntegerOverflow=on
  PaO2 : Outport
  tag scope: PAO2_delayIC=global, PaO2firstIC=global, PaO2secondIC=global
  wires:
  1/(T1*T2)/1 -> Integrator/1
  Sum/1 -> 1/(T1*T2)/1
  Integrator/1 -> Integrator1/1, T1+T2/1, [PaO2firstIC]
  Integrator1/1 -> [PaO2secondIC], Sum/2, PaO2/1
  T1+T2/1 -> Sum/3
  Product1/1 -> PAO2 delay/2
  PAO2/1 -> PAO2 delay/1
  PAO2 delay/1 -> [PAO2_delayIC], Sum/1
  Lung-Chemoreceptor Delay Volume/1 -> Product1/1
  Q/1 -> Product1/2

== system Respiratory/Gas Exchange/DEAD SPACE/CO2 DEAD SPACE ==
  PACO2 : Inport
  Flow : Inport  Port=2
  CO2 Partial Pressure : Subsystem  mask{begin_time=t_CO2_start, end_time=t_CO2_start+t_CO2_duration, init_value=PICO2, final_value=PICO2+PICO2_change}
      mask prompts: begin_time "pulse begin"; end_time "pulse end"; init_value "initial value"; final_value "final value"
      mask Display: disp('pulse')
  Pd(1)CO2 : Subsystem
  Pd(2)CO2 : Subsystem
  Pd(3)CO2 : Subsystem
  Pd(4)CO2 : Subsystem
  Pd(5)CO2 : Subsystem
  Pd5CO2 : Outport
  wires:
  Pd(4)CO2/1(Pd(4)CO2) -> Pd(3)CO2/3(Pd(4)CO2), Pd(5)CO2/1(Pd(4)CO2)
  Pd(3)CO2/1(Pd(3)CO2) -> Pd(4)CO2/1(Pd(3)CO2), Pd(2)CO2/3(Pd(3)CO2)
  Pd(2)CO2/1(Pd(2)CO2) -> Pd(3)CO2/1(Pd(2)CO2), Pd(1)CO2/3(Pd(2)CO2)
  Pd(1)CO2/1(Pd(1)CO2) -> Pd(2)CO2/1(Pd(1)CO2)
  Flow/1 -> Pd(1)CO2/2(Flow), Pd(2)CO2/2(Flow), Pd(4)CO2/2(Flow), Pd(5)CO2/2(Flow), Pd(3)CO2/2(Flow)
  PACO2/1 -> Pd(5)CO2/3(PACO2)
  Pd(5)CO2/1(Pd(5)CO2) -> Pd5CO2/1, Pd(4)CO2/3(Pd(5)CO2)
  CO2 Partial Pressure/1(Out1) -> Pd(1)CO2/1(PICO2)

== system Respiratory/Gas Exchange/DEAD SPACE/O2 DEAD SPACE ==
  Flow : Inport
  PAO2 : Inport  Port=2
  O2 Partial Pressure : Subsystem  mask{begin_time=t_O2_start, end_time=t_O2_start+t_O2_duration, init_value=PIO2, final_value=PIO2+PIO2_change}
      mask prompts: begin_time "pulse begin"; end_time "pulse end"; init_value "initial value"; final_value "final value"
      mask Display: disp('pulse')
  Pd(1)O2 : Subsystem
  Pd(2)O2 : Subsystem
  Pd(3)O2 : Subsystem
  Pd(4)O2 : Subsystem
  Pd(5)O2 : Subsystem
  Pd5O2 : Outport
  wires:
  Pd(4)O2/1(Pd(4)O2) -> Pd(3)O2/3(Pd(4)O2), Pd(5)O2/1(Pd(4)O2)
  Pd(3)O2/1(Pd(3)O2) -> Pd(4)O2/1(Pd(3)O2), Pd(2)O2/3(Pd(3)O2)
  Pd(2)O2/1(Pd(2)O2) -> Pd(3)O2/1(Pd(2)O2), Pd(1)O2/3(Pd(2)O2)
  Pd(1)O2/1(Pd(1)O2) -> Pd(2)O2/1(Pd(1)O2)
  PAO2/1 -> Pd(5)O2/3(PAO2)
  Flow/1 -> Pd(4)O2/2(Flow), Pd(5)O2/2(Flow), Pd(2)O2/2(Flow), Pd(1)O2/2(Flow), Pd(3)O2/2(Flow)
  Pd(5)O2/1(Pd(5)O2) -> Pd5O2/1, Pd(4)O2/3(Pd(5)O2)
  O2 Partial Pressure/1(Out1) -> Pd(1)O2/1(PIO2)
